simulink model "sim_RBF_Neural_Robot_Controller_Design_with_Sliding"  (R2023a)
settings: Solver=VariableStepAuto  StartTime=0.0  StopTime=40  RelTol=1e-3
settings Model: Creator=ACCENT  LastModifiedBy=ACCENT

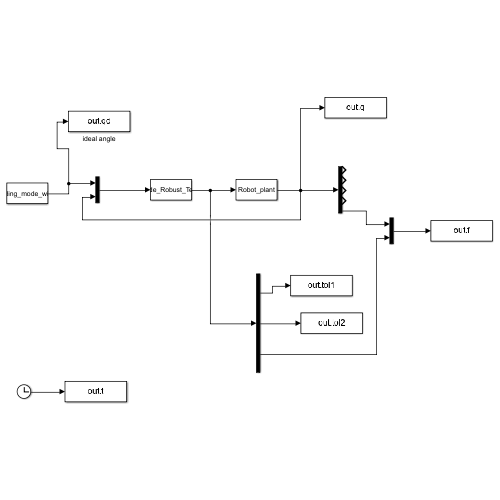
[thumbnail: Simulink's stored preview of the top-level diagram]
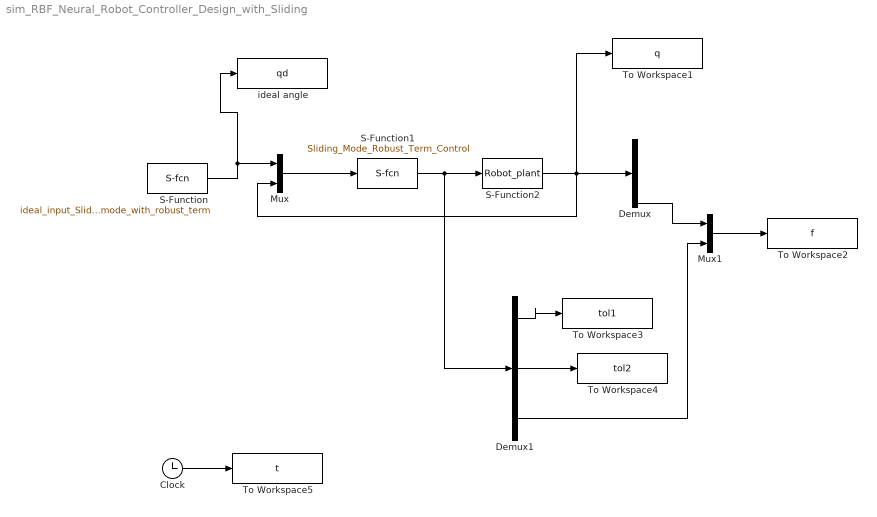
== system sim_RBF_Neural_Robot_Controller_Design_with_Sliding ==
  Clock : Clock
      settings: Decimation=40
  Demux : Demux  Outputs=5
  Demux1 : Demux  Outputs=3
  Mux : Mux  Inputs=2
  Mux1 : Mux  Inputs=2
  S-Function : S-Function  FunctionName=ideal_input_Sliding_mode_with_robust_term  SFunctionDeploymentMode=off  EnableBusSupport=off
  S-Function1 : S-Function  FunctionName=Sliding_Mode_Robust_Term_Control  SFunctionDeploymentMode=off  EnableBusSupport=off
  S-Function2 : S-Function  FunctionName=Robot_plant  SFunctionDeploymentMode=off  EnableBusSupport=off
  To Workspace1 : ToWorkspace  VariableName=q  SampleTime=-1
  To Workspace2 : ToWorkspace  VariableName=f  SampleTime=-1
  To Workspace3 : ToWorkspace  VariableName=tol1  SampleTime=-1
  To Workspace4 : ToWorkspace  VariableName=tol2  SampleTime=-1
  To Workspace5 : ToWorkspace  VariableName=t  SampleTime=-1
  ideal angle : ToWorkspace  VariableName=qd  SampleTime=-1
  wires:
  Clock/1 -> To Workspace5/1
  Demux/5 -> Mux1/1
  S-Function/1 -> ideal angle/1, Mux/1
  Mux/1 -> S-Function1/1
  S-Function1/1 -> Demux1/1, S-Function2/1
  S-Function2/1 -> Mux/2, To Workspace1/1, Demux/1
  Demux1/3 -> Mux1/2
  Demux1/2 -> To Workspace4/1
  Demux1/1 -> To Workspace3/1
  Mux1/1 -> To Workspace2/1
